simulink model "Fzgsym"  (R2022a)
settings: Solver=VariableStepAuto  StartTime=0.0  StopTime=30  RelTol=1e-3
values from neighbouring files (symbols this model uses):
  g = 9.81    [Energiebedarf_single.m]
  m = 1500    [Energiebedarf_single.m]
undefined symbols (not defined in the file or in its folder): air_temp, Bremsdruck_max, disk_abore, Drehmoment, Drehzahl, efficiency, l_CG_rear, mass_veh, mu_kinetic, num_pads, Rm, trq_eff
libraries: simulink x7, autolibshared x7, autolibmappedmotor x4, autolibutils x1, autolibdatasheetbattery x1
(part 3 of 3)

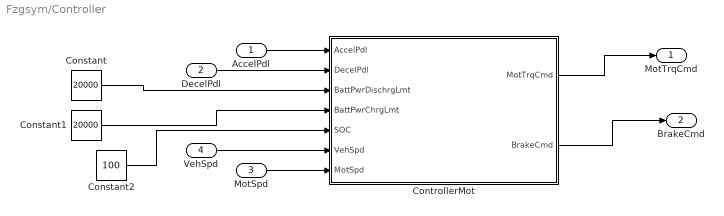
== system Fzgsym/Controller ==
  AccelPdl : Inport
  DecelPdl : Inport  Port=2
  MotSpd : Inport  Port=3
  VehSpd : Inport  Port=4
  Constant : Constant  Value=20000
  Constant1 : Constant  Value=20000
  Constant2 : Constant  Value=100
  ControllerMot : Subsystem
  MotTrqCmd : Outport
  BrakeCmd : Outport  Port=2
  wires:
  MotSpd/1 -> ControllerMot/7(MotSpd)
  AccelPdl/1 -> ControllerMot/1(AccelPdl)
  VehSpd/1 -> ControllerMot/6(VehSpd)
  DecelPdl/1 -> ControllerMot/2(DecelPdl)
  ControllerMot/1(MotTrqCmd) -> MotTrqCmd/1
  ControllerMot/2(BrakeCmd) -> BrakeCmd/1
  Constant2/1 -> ControllerMot/5(SOC)
  Constant1/1 -> ControllerMot/4(BattPwrChrgLmt)
  Constant/1 -> ControllerMot/3(BattPwrDischrgLmt)

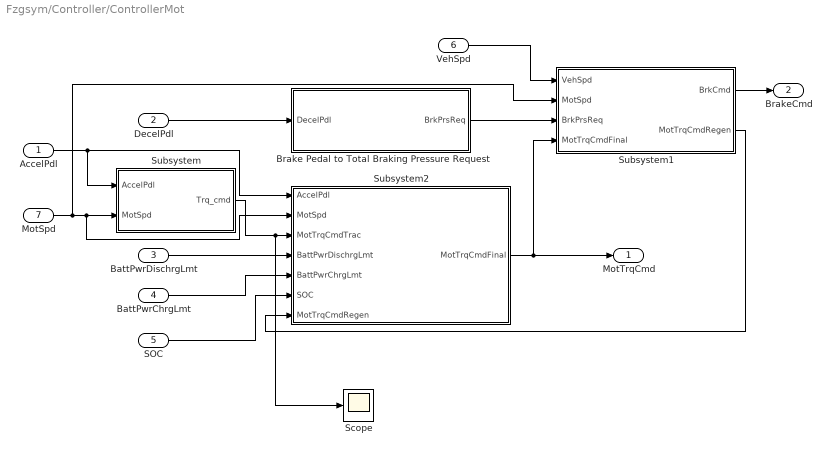
== system Fzgsym/Controller/ControllerMot ==
  AccelPdl : Inport
  DecelPdl : Inport  Port=2
  BattPwrDischrgLmt : Inport  Port=3
  BattPwrChrgLmt : Inport  Port=4
  SOC : Inport  Port=5
  VehSpd : Inport  Port=6
  MotSpd : Inport  Port=7
  Brake Pedal to Total Braking Pressure Request : Subsystem
  Scope : Scope
  Subsystem : Subsystem
  Subsystem1 : Subsystem
  Subsystem2 : Subsystem
  MotTrqCmd : Outport
  BrakeCmd : Outport  Port=2
  wires:
  Subsystem1/1(BrkCmd) -> BrakeCmd/1
  Subsystem1/2(MotTrqCmdRegen) -> Subsystem2/7(MotTrqCmdRegen)
  BattPwrChrgLmt/1 -> Subsystem2/5(BattPwrChrgLmt)
  VehSpd/1 -> Subsystem1/1(VehSpd)
  MotSpd/1 -> Subsystem/2(MotSpd), Subsystem2/2(MotSpd), Subsystem1/2(MotSpd)
  SOC/1 -> Subsystem2/6(SOC)
  AccelPdl/1 -> Subsystem2/1(AccelPdl), Subsystem/1(AccelPdl)
  BattPwrDischrgLmt/1 -> Subsystem2/4(BattPwrDischrgLmt)
  Subsystem/1(Trq_cmd) -> Scope/1, Subsystem2/3(MotTrqCmdTrac)
  Subsystem2/1(MotTrqCmdFinal) -> MotTrqCmd/1, Subsystem1/4(MotTrqCmdFinal)
  Brake Pedal to Total Braking Pressure Request/1(BrkPrsReq) -> Subsystem1/3(BrkPrsReq)
  DecelPdl/1 -> Brake Pedal to Total Braking Pressure Request/1(DecelPdl)

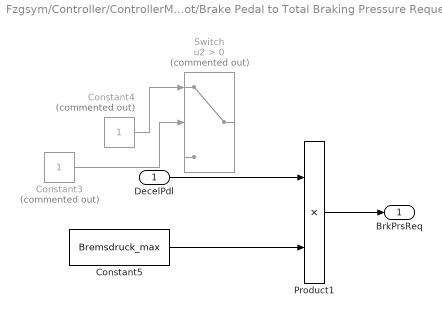
== system Fzgsym/Controller/ControllerMot/Brake Pedal to Total Braking Pressure Request ==
  DecelPdl : Inport
  Constant3 : Constant  Commented=on
  Constant4 : Constant  Commented=on
  Constant5 : Constant  Value=Bremsdruck_max
  Product1 : Product
  Switch : Switch  Commented=on  Criteria=u2 > Threshold  SaturateOnIntegerOverflow=off  InputSameDT=off
  BrkPrsReq : Outport
  wires:
  DecelPdl/1 -> Product1/1
  Constant3/1 -> Switch/2
  Constant5/1 -> Product1/2
  Constant4/1 -> Switch/1
  Product1/1 -> BrkPrsReq/1

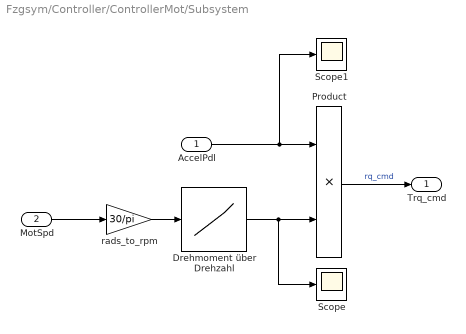
== system Fzgsym/Controller/ControllerMot/Subsystem ==
  AccelPdl : Inport
  MotSpd : Inport  Port=2
  Drehmoment über Drehzahl : Lookup_n-D  NumberOfTableDimensions=1  BreakpointsForDimension1=Drehzahl  BreakpointsForDimension3=[5, 7]  Table=Drehmoment*4  InternalRulePriority=Speed  RndMeth=Simplest
  Product : Product
  Scope : Scope
  Scope1 : Scope
  rads_to_rpm : Gain  Gain=30/pi
  Trq_cmd : Outport
  wires:
  Product/1 -> Trq_cmd/1  "rq_cmd"
  AccelPdl/1 -> Scope1/1, Product/1
  rads_to_rpm/1 -> Drehmoment über Drehzahl/1
  Drehmoment über Drehzahl/1 -> Scope/1, Product/2
  MotSpd/1 -> rads_to_rpm/1

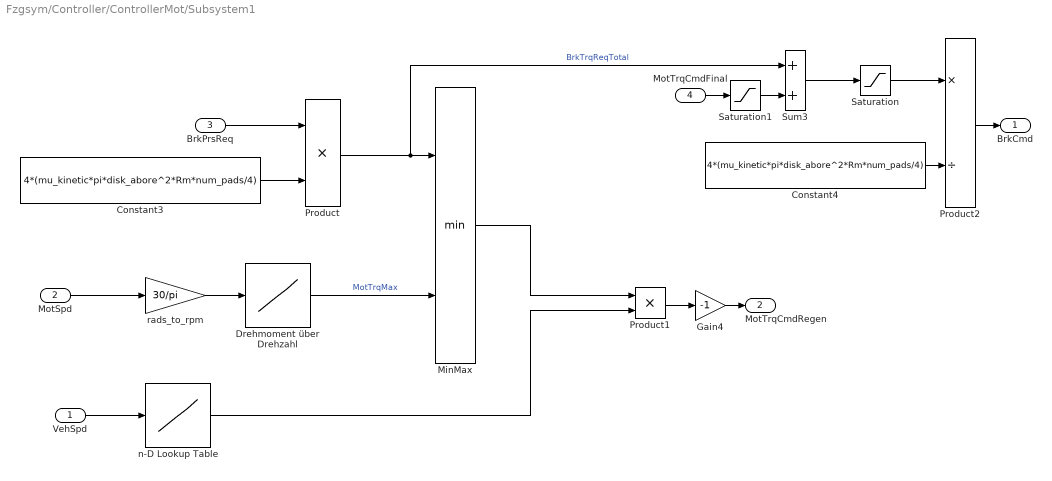
== system Fzgsym/Controller/ControllerMot/Subsystem1 ==
  VehSpd : Inport
  MotSpd : Inport  Port=2
  BrkPrsReq : Inport  Port=3
  MotTrqCmdFinal : Inport  Port=4
  Constant3 : Constant  Value=4*(mu_kinetic*pi*disk_abore^2*Rm*num_pads/4)
  Constant4 : Constant  Value=4*(mu_kinetic*pi*disk_abore^2*Rm*num_pads/4)
  Drehmoment über Drehzahl : Lookup_n-D  NumberOfTableDimensions=1  BreakpointsForDimension1=Drehzahl  BreakpointsForDimension3=[5, 7]  Table=Drehmoment  InternalRulePriority=Speed  RndMeth=Simplest
  Gain4 : Gain  Gain=-1
  MinMax : MinMax  Inputs=2
  Product : Product
  Product1 : Product
  Product2 : Product  Inputs=*/
  Saturation : Saturate  UpperLimit=inf  LowerLimit=0
  Saturation1 : Saturate  UpperLimit=0  LowerLimit=-inf
  Sum3 : Sum
  n-D Lookup Table : Lookup_n-D  NumberOfTableDimensions=1  BreakpointsForDimension1=[5 9]  BreakpointsForDimension3=[5, 7]  Table=[0 1]  InternalRulePriority=Speed  RndMeth=Simplest
  rads_to_rpm : Gain  Gain=30/pi
  BrkCmd : Outport
  MotTrqCmdRegen : Outport  Port=2
  wires:
  Sum3/1 -> Saturation/1
  MinMax/1 -> Product1/1
  BrkPrsReq/1 -> Product/1
  Constant4/1 -> Product2/2
  Product1/1 -> Gain4/1
  MotSpd/1 -> rads_to_rpm/1
  Drehmoment über Drehzahl/1 -> MinMax/2  "MotTrqMax"
  Product/1 -> Sum3/1, MinMax/1  "BrkTrqReqTotal"
  n-D Lookup Table/1 -> Product1/2
  Saturation/1 -> Product2/1
  Constant3/1 -> Product/2
  rads_to_rpm/1 -> Drehmoment über Drehzahl/1
  VehSpd/1 -> n-D Lookup Table/1
  Gain4/1 -> MotTrqCmdRegen/1
  MotTrqCmdFinal/1 -> Saturation1/1
  Product2/1 -> BrkCmd/1
  Saturation1/1 -> Sum3/2

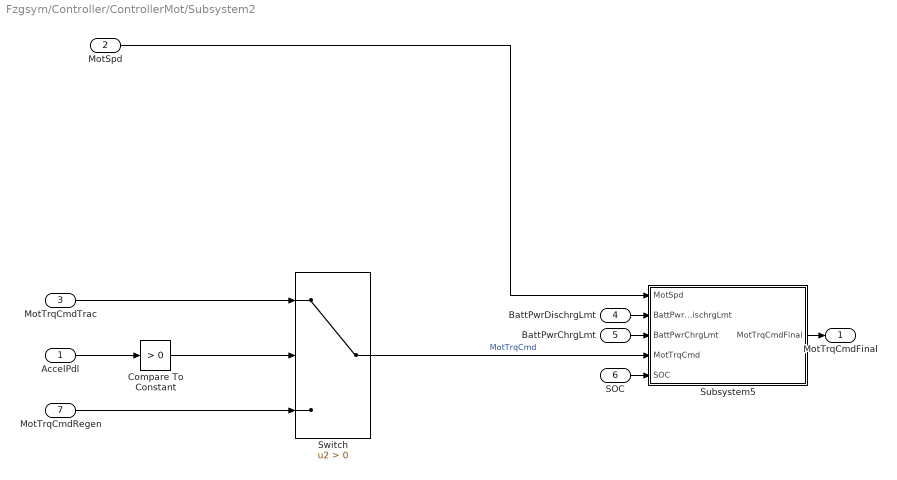
== system Fzgsym/Controller/ControllerMot/Subsystem2 ==
  AccelPdl : Inport
  MotSpd : Inport  Port=2
  MotTrqCmdTrac : Inport  Port=3
  BattPwrDischrgLmt : Inport  Port=4
  BattPwrChrgLmt : Inport  Port=5
  SOC : Inport  Port=6
  MotTrqCmdRegen : Inport  Port=7
  Compare To Constant : simulink/Logic and Bit Operations/Compare To Constant  relop=>  const=0  OutDataTypeStr=boolean
  Subsystem5 : Subsystem
  Switch : Switch  Criteria=u2 > Threshold  SaturateOnIntegerOverflow=off  InputSameDT=off
  MotTrqCmdFinal : Outport
  wires:
  Subsystem5/1(MotTrqCmdFinal) -> MotTrqCmdFinal/1
  SOC/1 -> Subsystem5/5(SOC)
  Switch/1 -> Subsystem5/4(MotTrqCmd)  "MotTrqCmd"
  Compare To Constant/1 -> Switch/2
  BattPwrDischrgLmt/1 -> Subsystem5/2(BattPwrDischrgLmt)
  AccelPdl/1 -> Compare To Constant/1
  BattPwrChrgLmt/1 -> Subsystem5/3(BattPwrChrgLmt)
  MotSpd/1 -> Subsystem5/1(MotSpd)
  MotTrqCmdRegen/1 -> Switch/3
  MotTrqCmdTrac/1 -> Switch/1

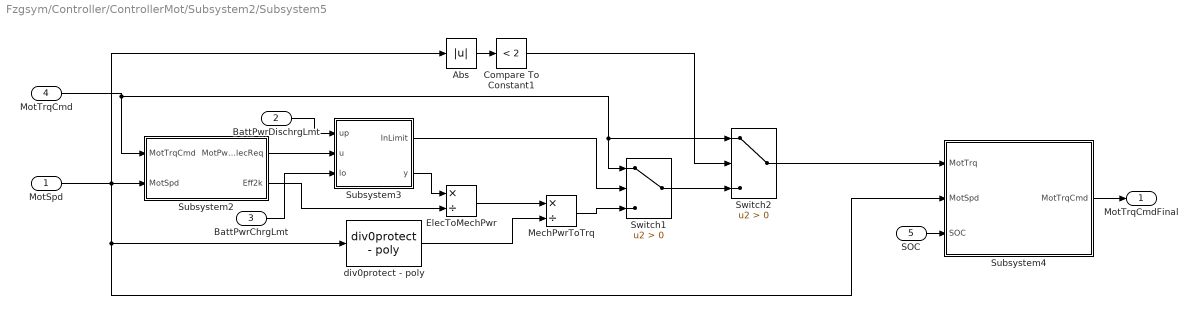
== system Fzgsym/Controller/ControllerMot/Subsystem2/Subsystem5 ==
  MotSpd : Inport
  BattPwrDischrgLmt : Inport  Port=2
  BattPwrChrgLmt : Inport  Port=3
  MotTrqCmd : Inport  Port=4
  SOC : Inport  Port=5
  Abs : Abs  SaturateOnIntegerOverflow=off
  Compare To Constant1 : simulink/Logic and Bit Operations/Compare To Constant  relop=<  const=2  OutDataTypeStr=boolean
  ElecToMechPwr : Product  Inputs=*/
  MechPwrToTrq : Product  Inputs=*/
  Subsystem2 : Subsystem
  Subsystem3 : Subsystem
  Subsystem4 : Subsystem
  Switch1 : Switch  Criteria=u2 > Threshold  SaturateOnIntegerOverflow=off  InputSameDT=off
  Switch2 : Switch  Criteria=u2 > Threshold  SaturateOnIntegerOverflow=off  InputSameDT=off
  div0protect - poly : autolibutils/div0protect - poly  thresh=2  ZeroCross1=off  aMode=aMode
      settings: SourceProductBaseCode=PW,DR,MT,VE
  MotTrqCmdFinal : Outport
  wires:
  Subsystem2/1(MotPwrElecReq) -> Subsystem3/2(u)
  MotSpd/1 -> Subsystem4/2(MotSpd), div0protect - poly/1, Abs/1, Subsystem2/2(MotSpd)
  BattPwrDischrgLmt/1 -> Subsystem3/1(up)
  MotTrqCmd/1 -> Subsystem2/1(MotTrqCmd), Switch1/1, Switch2/1
  div0protect - poly/1 -> MechPwrToTrq/2
  MechPwrToTrq/1 -> Switch1/3
  Switch2/1 -> Subsystem4/1(MotTrq)
  Subsystem2/2(Eff2k) -> ElecToMechPwr/2
  Subsystem3/1(InLimit) -> Switch1/2
  ElecToMechPwr/1 -> MechPwrToTrq/1
  Compare To Constant1/1 -> Switch2/2
  SOC/1 -> Subsystem4/3(SOC)
  Abs/1 -> Compare To Constant1/1
  Switch1/1 -> Switch2/3
  Subsystem3/2(y) -> ElecToMechPwr/1
  BattPwrChrgLmt/1 -> Subsystem3/3(lo)
  Subsystem4/1(MotTrqCmd) -> MotTrqCmdFinal/1

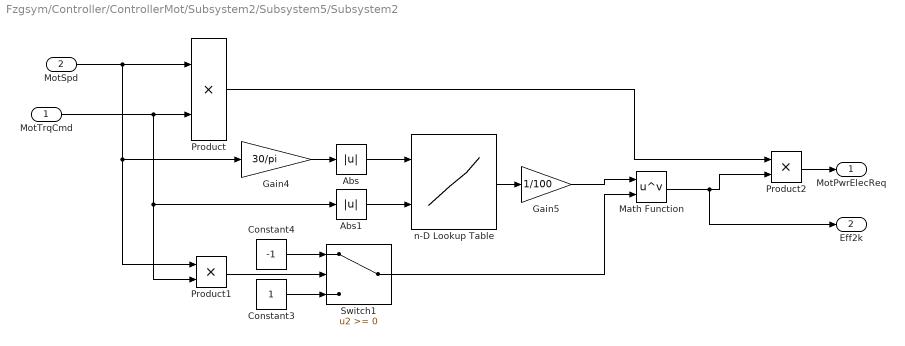
== system Fzgsym/Controller/ControllerMot/Subsystem2/Subsystem5/Subsystem2 ==
  MotTrqCmd : Inport
  MotSpd : Inport  Port=2
  Abs : Abs  SaturateOnIntegerOverflow=off
  Abs1 : Abs  SaturateOnIntegerOverflow=off
  Constant3 : Constant
  Constant4 : Constant  Value=-1
  Gain4 : Gain  Gain=30/pi
  Gain5 : Gain  Gain=1/100
  Math Function : Math  Operator=pow  SignedPower=on  OutputSignalType=real
  Product : Product
  Product1 : Product
  Product2 : Product
  Switch1 : Switch  SaturateOnIntegerOverflow=off  InputSameDT=off
  n-D Lookup Table : Lookup_n-D  BreakpointsForDimension1=Drehzahl  BreakpointsForDimension2=trq_eff  BreakpointsForDimension3=[5, 7]  Table=efficiency  InternalRulePriority=Speed  RndMeth=Simplest
      settings: InputPortMap=u0,u1
  MotPwrElecReq : Outport
  Eff2k : Outport  Port=2
  wires:
  Constant4/1 -> Switch1/1
  Switch1/1 -> Math Function/2
  Product1/1 -> Switch1/2
  Constant3/1 -> Switch1/3
  Gain5/1 -> Math Function/1
  Product/1 -> Product2/1
  Abs1/1 -> n-D Lookup Table/2
  MotTrqCmd/1 -> Abs1/1, Product1/2, Product/2
  MotSpd/1 -> Product/1, Product1/1, Gain4/1
  Abs/1 -> n-D Lookup Table/1
  n-D Lookup Table/1 -> Gain5/1
  Gain4/1 -> Abs/1
  Math Function/1 -> Eff2k/1, Product2/2
  Product2/1 -> MotPwrElecReq/1

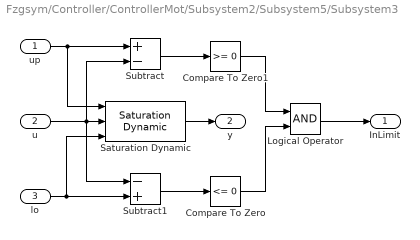
== system Fzgsym/Controller/ControllerMot/Subsystem2/Subsystem5/Subsystem3 ==
  up : Inport
  u : Inport  Port=2
  lo : Inport  Port=3
  Compare To Zero : simulink/Logic and Bit Operations/Compare To Zero  relop=<=  OutDataTypeStr=boolean
  Compare To Zero1 : simulink/Logic and Bit Operations/Compare To Zero  relop=>=  OutDataTypeStr=boolean
  Logical Operator : Logic  AllPortsSameDT=off  OutDataTypeStr=boolean
  Saturation Dynamic : simulink/Discontinuities/Saturation Dynamic  OutMin=[]  OutMax=[]  OutDataTypeStr=Inherit: Same as second input  OutDataType=fixdt(1, 16)  OutScaling=2^-10  DoSatur=off
  Subtract : Sum  Inputs=+-
  Subtract1 : Sum  Inputs=-+
  InLimit : Outport
  y : Outport  Port=2
  wires:
  Subtract1/1 -> Compare To Zero/1
  Logical Operator/1 -> InLimit/1
  Subtract/1 -> Compare To Zero1/1
  Compare To Zero1/1 -> Logical Operator/1
  Compare To Zero/1 -> Logical Operator/2
  lo/1 -> Saturation Dynamic/3, Subtract1/2
  up/1 -> Saturation Dynamic/1, Subtract/1
  u/1 -> Subtract1/1, Subtract/2, Saturation Dynamic/2
  Saturation Dynamic/1 -> y/1

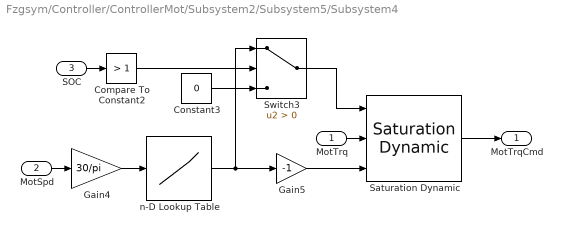
== system Fzgsym/Controller/ControllerMot/Subsystem2/Subsystem5/Subsystem4 ==
  MotTrq : Inport
  MotSpd : Inport  Port=2
  SOC : Inport  Port=3
  Compare To Constant2 : simulink/Logic and Bit Operations/Compare To Constant  relop=>  const=1  OutDataTypeStr=boolean
  Constant3 : Constant  Value=0
  Gain4 : Gain  Gain=30/pi
  Gain5 : Gain  Gain=-1
  Saturation Dynamic : simulink/Discontinuities/Saturation Dynamic  OutMin=[]  OutMax=[]  OutDataTypeStr=Inherit: Same as second input  OutDataType=fixdt(1, 16)  OutScaling=2^-10  DoSatur=off
  Switch3 : Switch  Criteria=u2 > Threshold  SaturateOnIntegerOverflow=off  InputSameDT=off
  n-D Lookup Table : Lookup_n-D  NumberOfTableDimensions=1  BreakpointsForDimension1=Drehzahl  BreakpointsForDimension3=[5, 7]  Table=Drehmoment  InternalRulePriority=Speed  RndMeth=Simplest
  MotTrqCmd : Outport
  wires:
  n-D Lookup Table/1 -> Gain5/1, Switch3/1
  Constant3/1 -> Switch3/3
  MotSpd/1 -> Gain4/1
  Switch3/1 -> Saturation Dynamic/1
  Compare To Constant2/1 -> Switch3/2
  Gain4/1 -> n-D Lookup Table/1
  Gain5/1 -> Saturation Dynamic/3
  SOC/1 -> Compare To Constant2/1
  Saturation Dynamic/1 -> MotTrqCmd/1
  MotTrq/1 -> Saturation Dynamic/2
